simulink model "detect_threshold"  (R2014a)
settings: Solver=FixedStepDiscrete  StartTime=0.0  StopTime=10.0  RelTol=1e-3
model workspace (MAT data in the model file):
  Fs = 48000
libraries: simulink x6, dspstat3 x2
settings Model: Creator=User  LastModifiedBy=User
settings OptimizationCC: InlineParams=on

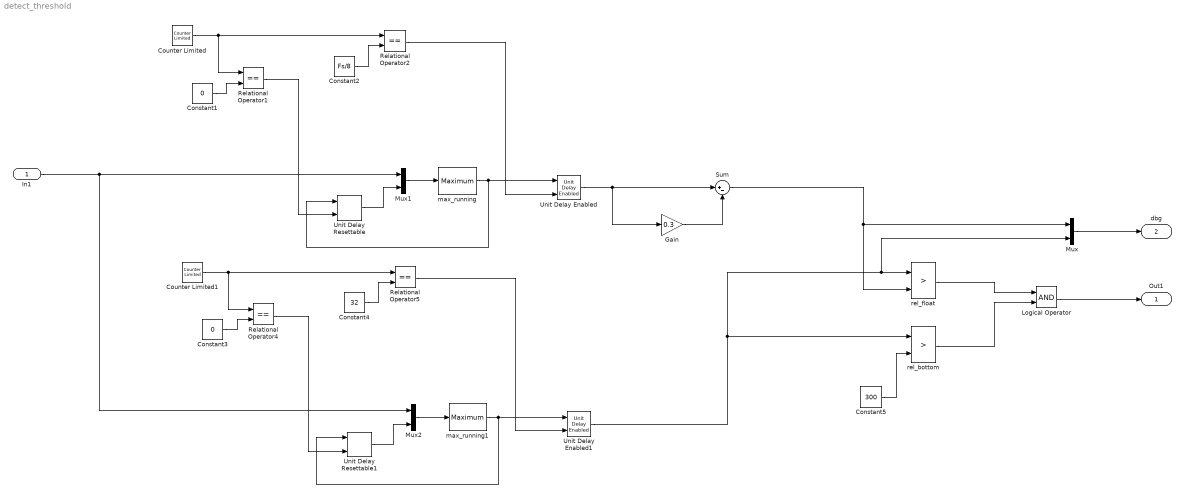
== system detect_threshold ==
  In1 : Inport  OutDataTypeStr=fixdt(1,16,0)
  Constant1 : Constant  Value=0  OutDataTypeStr=Inherit: Inherit via back propagation
  Constant2 : Constant  Value=Fs/8  OutDataTypeStr=Inherit: Inherit via back propagation
  Constant3 : Constant  Value=0  OutDataTypeStr=Inherit: Inherit via back propagation
  Constant4 : Constant  Value=32  OutDataTypeStr=Inherit: Inherit via back propagation
  Constant5 : Constant  Value=300  OutDataTypeStr=Inherit: Inherit via back propagation
  Counter Limited : simulink/Sources/Counter Limited  uplimit=Fs/8  tsamp=-1
  Counter Limited1 : simulink/Sources/Counter Limited  uplimit=32  tsamp=-1
  Gain : Gain  Gain=0.3  OutDataTypeStr=fixdt(1,16,0)
  Logical Operator : Logic  AllPortsSameDT=off  OutDataTypeStr=boolean
  Mux : Mux  Inputs=2
  Mux1 : Mux  Inputs=2
  Mux2 : Mux  Inputs=2
  Relational Operator{1..2,4..5} (4 alike) : RelationalOperator  Operator===  OutDataTypeStr=boolean
  Sum : Sum  Inputs=|+-  AccumDataTypeStr=fixdt(1,16,0)
  Unit Delay Enabled : simulink/Additional Math & Discrete/Additional Discrete/Unit Delay Enabled  vinit=600  tsamp=-1
  Unit Delay Enabled1 : simulink/Additional Math & Discrete/Additional Discrete/Unit Delay Enabled  vinit=600  tsamp=-1
  Unit Delay Resettable : simulink/Additional Math & Discrete/Additional Discrete/Unit Delay Resettable  vinit=0  tsamp=-1
  Unit Delay Resettable1 : simulink/Additional Math & Discrete/Additional Discrete/Unit Delay Resettable  vinit=0  tsamp=-1
  max_running : dspstat3/Maximum  fcn=Value  reset=None  indexBase=One  operateOver=Each column  Dimension=1  colComp=on  operation=maximum  roiEnable=off  roiType=Rectangles  roiPortion=Entire ROI  roiOutput=Individual statistics for each ROI  roiFlag=off  accumDataTypeStr=Inherit: Same as product output  accumLastDataTypeStr=Inherit: Same as product output  roundingMode=Floor  overflowMode=off
  max_running1 : dspstat3/Maximum  fcn=Value  reset=None  indexBase=One  operateOver=Each column  Dimension=1  colComp=on  operation=maximum  roiEnable=off  roiType=Rectangles  roiPortion=Entire ROI  roiOutput=Individual statistics for each ROI  roiFlag=off  accumDataTypeStr=Inherit: Same as product output  accumLastDataTypeStr=Inherit: Same as product output  roundingMode=Floor  overflowMode=off
  rel_bottom : RelationalOperator  Operator=>  OutDataTypeStr=boolean
  rel_float : RelationalOperator  Operator=>  OutDataTypeStr=boolean
  Out1 : Outport
  dbg : Outport  Port=2
  wires:
  max_running/1 -> Unit Delay Enabled/1, Unit Delay Resettable/1
  Sum/1 -> Mux/1, rel_float/2
  Mux1/1 -> max_running/1
  Unit Delay Resettable/1 -> Mux1/2
  Logical Operator/1 -> Out1/1
  Counter Limited/1 -> Relational Operator1/1, Relational Operator2/1
  Constant1/1 -> Relational Operator1/2
  Constant2/1 -> Relational Operator2/2
  Relational Operator2/1 -> Unit Delay Enabled/2
  Relational Operator1/1 -> Unit Delay Resettable/2
  max_running1/1 -> Unit Delay Resettable1/1, Unit Delay Enabled1/1
  Mux2/1 -> max_running1/1
  Unit Delay Resettable1/1 -> Mux2/2
  Counter Limited1/1 -> Relational Operator5/1, Relational Operator4/1
  Constant3/1 -> Relational Operator4/2
  Constant4/1 -> Relational Operator5/2
  Relational Operator5/1 -> Unit Delay Enabled1/2
  Relational Operator4/1 -> Unit Delay Resettable1/2
  In1/1 -> Mux2/1, Mux1/1
  Unit Delay Enabled1/1 -> rel_bottom/1, Mux/2, rel_float/1
  Unit Delay Enabled/1 -> Gain/1, Sum/1
  Gain/1 -> Sum/2
  rel_bottom/1 -> Logical Operator/2
  rel_float/1 -> Logical Operator/1
  Constant5/1 -> rel_bottom/2
  Mux/1 -> dbg/1
